simulink model "code_gen"  (Simulink 7.5)
settings: Solver=FixedStepDiscrete  StartTime=0.0  StopTime=10.0  FixedStep=0.001  RelTol=1e-3
InitFcn:
  | boat_constants
values from neighbouring files (symbols this model uses):
  InitialPoint = 0    [boat_constants.m]    (also in l2plus.m)
  IPStar = 0    [boat_constants.m]    (also in l2plus.m)
  ISA_g = 9.815    [boat_constants.m]
  MaxDwnPthStar = 1    [boat_constants.m]    (also in l2plus.m)
  OC2max = 49999    [boat_constants.m]    (also in simulation_constants.m)
  switchDistance = 4    [boat_constants.m]    (also in l2plus.m)
  T_step = 0.01    [boat_constants.m]    (also in common.m)
  tanIntercept = tan( 45*pi/180 )    [boat_constants.m]    (also in l2plus.m)
  TStar = single(4.5)    [boat_constants.m]    (also in l2plus.m = single(2))
  Turn2Track = 0    [boat_constants.m]    (also in l2plus.m)
undefined symbols (not defined in the file or in its folder): buildAndCheckMessage, buildAndCheckSentence, DiscIntNeverNeededParam, ecan1_buffered_transmit_matlab, ecan1_init, getGpsMainData, getSensorData, u1, y1
libraries: simulink x49, dsPICdrivers x22, simulink_need_slupdate x6, microSimulink x4, aerolibconvert2 x3
(part 1 of 3)
settings Model: Creator=bwmairs  LastModifiedBy=bwmairs
settings OptimizationCC: InlineParams=on  InlineInvariantSignals=on  EnhancedBackFolding=on  ZeroExternalMemoryAtStartup=off  ZeroInternalMemoryAtStartup=off  NoFixptDivByZeroProtection=on  EfficientFloat2IntCast=on  OptimizeModelRefInitCode=on
settings DebuggingCC: ReadBeforeWriteMsg=EnableAllAsError  WriteAfterWriteMsg=EnableAllAsError  WriteAfterReadMsg=EnableAllAsError  IntegerOverflowMsg=error  UniqueDataStoreMsg=error
settings HardwareCC: ProdBitPerInt=16  ProdIntDivRoundTo=Zero  ProdEndianess=LittleEndian  ProdWordSize=16  ProdHWDeviceType=16-bit Generic
settings RTWCC: SystemTargetFile=dspic.tlc  TemplateMakefile=dspic_pic30_gcc.tmf  PostCodeGenCommand=dsPIC_Compile()  Description=Embedded Target for Microchip dsPIC (real-time)  ProcessScript=dspic_make_rtw_hook  RTWCompilerOptimization=On
settings RTWCC: CustomSource=|
  | ../../../../ecan/cBuffer.c
  | ../../../../ecan/ecanFunctions.c
  | clib/gps.c
  | clib/sbrk.c
  | clib/commProtocol.c
settings CodeAppCC: IgnoreCustomStorageClasses=off
settings STFCustomTargetCC: IncludeMdlTerminateFcn=off  CombineOutputUpdateFcns=on  SuppressErrorStatus=on  ERTCustomFileBanners=on  SupportNonFinite=off  SupportContinuousTime=off  SupportNonInlinedSFcns=off  SystemTargetFile=dspic.tlc
settings ERTTargetCC: MultiwordLength=2048  ParMdlRefBuildCompliant=off  CompOptLevelCompliant=off  IncludeMdlTerminateFcn=off  SuppressErrorStatus=on  ERTFirstTimeCompliant=off  SupportNonFinite=off  ModelStepFunctionPrototypeControlCompliant=off  CPPClassGenCompliant=off  ExtModeMexFile=noextcomm  InlinedParameterPlacement=NonHierarchical  ERTSrcFileBannerTemplate=dsPIC_code_template.cgt  ERTHdrFileBannerTemplate=dsPIC_code_template.cgt  ERTDataSrcFileTemplate=dsPIC_code_template.cgt  ERTDataHdrFileTemplate=dsPIC_code_template.cgt  ERTCustomFileTemplate=dsPIC_main.tlc
settings CustomProperty: DataType=string  Value=C:\PROGRA~1\MATLAB\R2010a\bin\win32\gmake

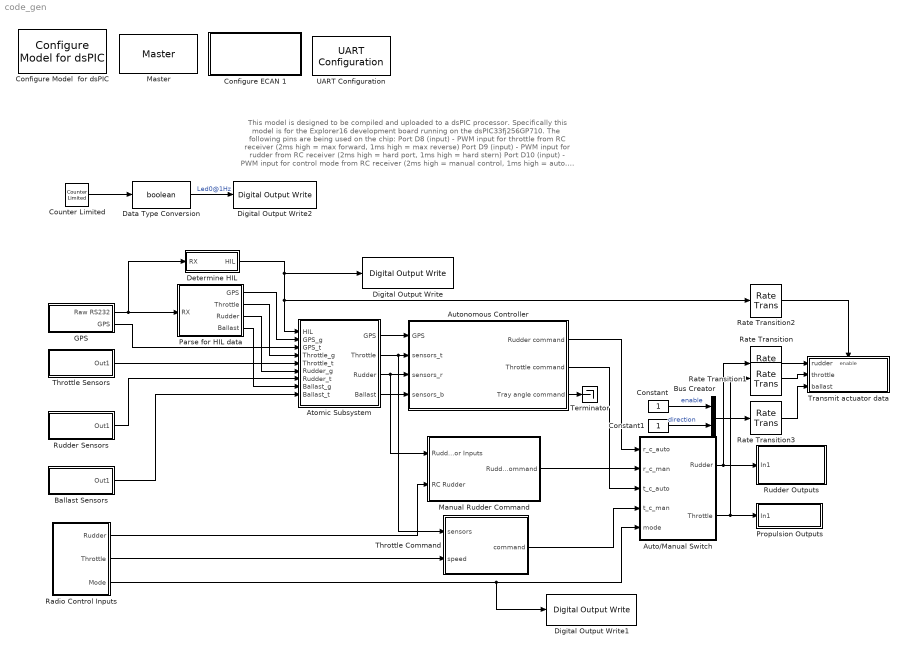
== system code_gen ==
  note: This model is designed to be compiled and uploaded to a dsPIC processor.
      | Specifically this model is for the Explorer16 development board running on
      | the dsPIC33fj256GP710. The following pins are being used on the chip:
      | Port D8 (input) - PWM input for throttle from RC receiver (2ms high = max forward, 1ms high = max reverse)
      | Port D9 (input) - PWM input for rudder from RC receiver (2ms high = hard port, 1ms high = hard stern)
      | Port D10 (input) - PWM input for control mode from RC receiver (2ms high = manual control, 1ms high = auto. control)
      | Port F3 (input) - Port hall effect sensor
      | Port G3 (input) - Starboard hall effect sensor
      | Port B0 (input) - Potentiometer measuring position for the rudder
      | Port OC2/RD1 (output) - Step output for the rudder driver board
      | Port G9 (output) - Enable output for the rudder driver board, wired low
      | Port D5 (output) - Direction output for the rudder driver board (low = rudder turns to port)
      | Ports F0/1 (in/out) - Pins required for the ECAN1 peripheral. This is used for controlling the propeller motor.
      | Ports F4/5 (in/out) - Pins required for the UART2 peripheral. This is used for HIL data or GPS input.
      |
      | A failsafe has been implemented to detect the loss of an RC connection. It reduces propeller speed to zero and
      | disables rudder control.
      |
      | Switching between the autonomous controller and manual control involves using the landing gear channel. When
      | it's enabled, it's under autonomous control. This can only be changed when the RC transmitter is on and connected and
      | is never changed otherwise.
  Atomic Subsystem : Subsystem
  Auto/Manual Switch : Subsystem
  Autonomous Controller : Subsystem
  Ballast Sensors : Subsystem
  Bus Creator : BusCreator  Inputs=2
  Configure ECAN 1 : Subsystem  mask(Initialize ECAN 1){frame_setting=off, mode=Normal, dma_rx_chan=2, dma_tx_chan=0, baud=250000, ps1=8, pd=5, ps2=6, sjw=4, tq=20, triple_sample=on, dma_buf_size=6 buffers, rx_bufs=[], tx_bufs=[0], buf_0_tx_pri=Highest, buf_0_rte=No, buf_1_tx_pri=Highest, buf_1_rte=No, buf_2_tx_pri=Lowest, buf_2_rte=No, buf_3_tx_pri=Lowest, buf_3_rte=No, buf_4_tx_pri=Lowest, buf_4_rte=No, buf_5_tx_pri=Lowest, buf_5_rte=No, buf_6_tx_pri=Lowest, buf_6_rte=No, buf_7_tx_pri=Lowest, buf_7_rte=No, mask_0=0, mask_0_mide=Match std or ext, mask_1=0, mask_1_mide=Match std or ext, mask_2=0, mask_2_mide=Match std or ext, filters=[], filter_0=hex2dec('400'), filter_0_mask=0, filter_0_exide=Match only standard, filter_0_buf=1, filter_1=hex2dec('401'), filter_1_mask=0, filter_1_exide=Match only standard, filter_1_buf=2, filter_2=hex2dec('402'), filter_2_mask=0, filter_2_exide=Match only standard, filter_2_buf=3, filter_3=0, filter_3_mask=0, filter_3_exide=Match only standard, filter_3_buf=0, filter_4=0, filter_4_mask=0, filter_4_exide=Match only standard, filter_4_buf=0, filter_5=0, filter_5_mask=0, filter_5_exide=Match only standard, filter_5_buf=0, filter_6=0, filter_6_mask=0, filter_6_exide=Match only standard, filter_6_buf=0, filter_7=0, filter_7_mask=0, filter_7_exide=Match only standard, filter_7_buf=0, filter_8=0, filter_8_mask=0, filter_8_exide=Match only standard, filter_8_buf=0, filter_9=0, filter_9_mask=<empty>, filter_9_exide=Match only standard, filter_9_buf=0, filter_10=0, filter_10_mask=0, filter_10_exide=Match only standard, filter_10_buf=0, filter_11=0, filter_11_mask=0, filter_11_exide=Match only standard, filter_11_buf=0, filter_12=0, filter_12_mask=0, filter_12_exide=Match only standard, filter_12_buf=0, filter_13=0, filter_13_mask=0, filter_13_exide=Match only standard, filter_13_buf=0, filter_14=0, filter_14_mask=0, filter_14_exide=Match only standard, filter_14_buf=0, filter_15=0, filter_15_mask=0, filter_15_exide=Match only standard, filter_15_buf=0}
      mask prompts: frame_setting "Extended Frames (Standard if unchecked)"; dma_rx_chan "DMA Reception Channel"; dma_tx_chan "DMA Transmission Channel"; baud "Baud Rate (bps)"; ps1 "Phase Segment 1"; pd "Propagation Delay"; ps2 "Phase Segment 2"; sjw "Sync Jump Width"; tq "Time Quanta"; triple_sample "Triple-sample"; dma_buf_size "DMA Buffer Size"; rx_bufs "Reception Buffers"; tx_bufs "Transmission Buffers"; buf_0_tx_pri "Buffer 0 Transmission Priority"; buf_0_rte "Buffer 0 Remote Transmit Enable"; buf_1_tx_pri "Buffer 1 Transmission Priority"; buf_1_rte "Buffer 1 Remote Transmit Enable"; buf_2_tx_pri "Buffer 2 Transmission Priority"; buf_2_rte "Buffer 2 Remote Transmit Enable"; buf_3_tx_pri "Buffer 3 Transmission Priority"; buf_3_rte "Buffer 3 Remote Transmit Enable"; buf_4_tx_pri "Buffer 4 Transmission Priority"; buf_4_rte "Buffer 4 Remote Transmit Enable"; buf_5_tx_pri "Buffer 5 Transmission Priority"; buf_5_rte "Buffer 5 Remote Transmit Enable"; buf_6_tx_pri "Buffer 6 Transmission Priority"; buf_6_rte "Buffer 6 Remote Transmit Enable"; buf_7_tx_pri "Buffer 7 Transmission Priority"; buf_7_rte "Buffer 7 Remote Transmit Enable"; mask_0 "Mask 0"; mask_0_mide "Mask 0 Receive Mode"; mask_1 "Mask 1"; mask_1_mide "Mask 1 Receive Mode"; mask_2 "Mask 2"; mask_2_mide "Mask 2 Receive Mode"; filter_0 "Filter 0"; filter_0_mask "Filter 0 Mask"; filter_0_exide "Filter 0 Mode"; filter_0_buf "Filter 0 Buffer"; filter_1 "Filter 1"; filter_1_mask "Filter 1 Mask"; filter_1_exide "Filter 1 Mode"; filter_1_buf "Filter 1 Buffer"; filter_2 "Filter 2"; filter_2_mask "Filter 2 Mask"; filter_2_exide "Filter 2 Mode"; filter_2_buf "Filter 2 Buffer"; filter_3 "Filter 3"; filter_3_mask "Filter 3 Mask"; filter_3_exide "Filter 3 Mode"; filter_3_buf "Filter 3 Buffer"; filter_4 "Filter 4"; filter_4_mask "Filter 4 Mask"; filter_4_exide "Filter 4 Mode"; filter_4_buf "Filter 4 Buffer"; filter_5 "Filter 5"; filter_5_mask "Filter 5 Mask"; filter_5_exide "Filter 5 Mode"; filter_5_buf "Filter 5 Buffer"; filter_6 "Filter 6"; filter_6_mask "Filter 6 Mask"; filter_6_exide "Filter 6 Mode"; filter_6_buf "Filter 6 Buffer"; filter_7 "Filter 7"; filter_7_mask "Filter 7 Mask"; filter_7_exide "Filter 7 Mode"; filter_7_buf "Filter 7 Buffer"; filter_8 "Filter 8"; filter_8_mask "Filter 8 Mask"; filter_8_exide "Filter 8 Mode"; filter_8_buf "Filter 8 Buffer"; filter_9 "Filter 9"; filter_9_mask "Filter 9 Mask"; filter_9_exide "Filter 9 Mode"; filter_9_buf "Filter 9 Buffer"; filter_10 "Filter 10"; filter_10_mask "Filter 10 Mask"; filter_10_exide "Filter 10 Mode"; filter_10_buf "Filter 10 Buffer"; filter_11 "Filter 11"; filter_11_mask "Filter 11 Mask"; filter_11_exide "Filter 11 Mode"; filter_11_buf "Filter 11 Buffer"; filter_12 "Filter 12"; filter_12_mask "Filter 12 Mask"; filter_12_exide "Filter 12 Mode"; filter_12_buf "Filter 12 Buffer"; filter_13 "Filter 13"; filter_13_mask "Filter 13 Mask"; filter_13_exide "Filter 13 Mode"; filter_13_buf "Filter 13 Buffer"; filter_14 "Filter 14"; filter_14_mask "Filter 14 Mask"; filter_14_exide "Filter 14 Mode"; filter_14_buf "Filter 14 Buffer"; filter_15 "Filter 15"; filter_15_mask "Filter 15 Mask"; filter_15_exide "Filter 15 Mode"; filter_15_buf "Filter 15 Buffer"
      mask help: Initializes the ECAN 1 module on the dsPIC33f. Allows for configuration of almost all ECAN options to produce a usable system.
      mask init:
      | parameters = uint16(zeros(53,1));
      | 
      | %% Generate parameter 1
      | parameters(1) = frame_setting;
      | mode_id = 0;
      | switch mode
      |     case 'Disabled'
      |         mode_id = 1;
      |     case 'Loopback'
      |         mode_id = 2;
      |     case 'Listen only'
      |         mode_id = 3;
      |     case 'Listen all'
      |         mode_id = 7;
      | end
      | parameters(1) = bitor(parameters(1), bitshift(mode_id, 2));
      | parameters(1) = bitor(parameters(1), bitshift(dma_rx_chan, 5));
      | parameters(1) = bitor(parameters(1), bitshift(dma_tx_chan, 8));
      | 
      | %% Generate parameter 2
      | parameters(2) = baud / 100;
      | 
      | %% Generate parameter 3
      | h = find_system(bdroot(gcb),'FollowLinks','on','LookUnderMasks','all','Tag','dsPIC_MASTER');
      | fcy = 0;
      | if ~isempty(h)
      |     %OverrideFcy = strcmp(get_param(h{1},'OverrideFcy'),'on');
      |     %if (OverrideFcy == 1)
      |     %    fcy = str2num(get_param(h{1},'NewFcy'));     %% overridded fcy
      |     %else
      |         fcy = str2num(get_param(h{1},'fcy'));
      |     %end 
      | end
      | parameters(3) = fcy / 1000;
      | 
      | %% Generate parameter 4
      | parameters(4) = ps1 - 1;
      | parameters(4) = bitor(parameters(4), bitshift(pd - 1, 3));
      | parameters(4) = bitor(parameters(4), bitshift(ps2 - 1, 6));
      | parameters(4) = bitor(parameters(4), bitshift(sjw - 1, 9));
      | if triple_sample == 1
      |     parameters(4) = bitset(parameters(4),12);
      | end
      | 
      | %% Generate parameter 5
      | for k = 1:length(filters)
      |     parameters(5) = bitset(parameters(5),filters(k)+1);
      | end;
      | 
      | % Map filter mask values into proper values
      | filter_masks = [filter_0_mask; filter_1_mask; filter_2_mask; filter_3_mask; filter_4_mask; filter_5_mask; filter_6_mask; filter_7_mask; filter_8_mask; filter_9_mask; filter_10_mask; filter_11_mask; filter_12_mask; filter_13_mask; filter_14_mask; filter_15_mask;];
      | filter_masks = filter_masks - 2;
      | filter_masks(filter_masks == -1) = 3;
      | 
      | %% Generate parameters 6 and 7
      | for k = 1:length(filters);
      |     filter = filters(k) + 1;
      |     if filter < 9
      |         parameters(6) = bitor(parameters(6), bitshift(filter_masks(filter),2*(filter-1)));
      |     else
      |         parameters(7) = bitor(parameters(7), bitshift(filter_masks(filter),2*(filter-9)));
      |     end
      | end
      | 
      | % Generate parameters 8 and 9
      | parameters(8) = bitshift(bitand(mask_0,hex2dec('18000000')),-27); % EID17-16
      | parameters(8) = bitor(parameters(8), bitshift(bitand(mask_0,hex2dec('7FF')), 5)); % SID
      | parameters(8) = bitor(parameters(8), bitshift(mask_0_mide - 1, 3)); % MIDE
      | parameters(9) = bitshift(bitand(mask_0,hex2dec('7FFF800')),-11); % EID15-0
      | 
      | %% Generate parameters 10 and 11
      | parameters(10) = bitshift(bitand(mask_1,hex2dec('18000000')),-27); % EID17-16
      | parameters(10) = bitor(parameters(10), bitshift(bitand(mask_1,hex2dec('7FF')), 5)); % SID
      | parameters(10) = bitor(parameters(10), bitshift(mask_1_mide - 1, 3)); % MIDE
      | parameters(11) = bitshift(bitand(mask_1,hex2dec('7FFF800')),-11); % EID15-0
      | 
      | %% Generate parameters 12 and 13
      | parameters(12) = bitshift(bitand(mask_2,hex2dec('18000000')),-27); % EID17-16
      | parameters(12) = bitor(parameters(12), bitshift(bitand(mask_2,hex2dec('7FF')), 5)); % SID
      | parameters(12) = bitor(parameters(12), bitshift(mask_2_mide - 1, 3)); % MIDE
      | parameters(13) = bitshift(bitand(mask_2,hex2dec('7FFF800')),-11); % EID15-0
      | 
      | % Generate parameters 14-17
      | buf_priorities = [buf_0_tx_pri;buf_1_tx_pri;buf_2_tx_pri;buf_3_tx_pri;buf_4_tx_pri;buf_5_tx_pri;buf_6_tx_pri;buf_7_tx_pri] - 1;
      | buf_rtes = [buf_0_rte;buf_1_rte;buf_2_rte;buf_3_rte;buf_4_rte;buf_5_rte;buf_6_rte;buf_7_rte] - 1;
      | 
      | % Create a vector of chars to modify
      | regs = uint16(zeros(8,1));
      | 
      | % Go through all enabled transmission buffers setting appropriate bits
      | for b = 1:size(tx_bufs,1)
      |     
      |     index = tx_bufs(b) + 1;
      |     
      |     % Set transmission bit
      |     regs(index) = bitset(regs(index),8);
      | 
      |     % Set priority bits
      |     regs(index) = bitor(regs(index), buf_priorities(index));
      | 
      |     % Set remote transmit enable bits
      |     if buf_rtes(index) == 1
      |         regs(index) = bitset(regs(index),3);
      |     end
      | end
      | 
      | for b = 1:size(rx_bufs,1)
      |     
      |     index = rx_bufs(b) + 1;
      | 
      |     % Set priority bits
      |     regs(index) = bitor(regs(index), buf_priorities(index));
      | 
      |     % Set remote transmit enable bits
      |     if buf_rtes(index) == 1
      |         regs(index) = bitset(regs(index),3);
      |     end
      | end
      | 
      | % Map our matrix into registers
      | parameters(14) = bitor(bitshift(regs(2),8), regs(1));
      | parameters(15) = bitor(bitshift(regs(4),8), regs(3));
      | parameters(16) = bitor(bitshift(regs(6),8), regs(5));
      | parameters(17) = bitor(bitshift(regs(8),8), regs(7));
      | 
      | % Map the filter buffer values to corresponding bit values
      | filter_buffers = [filter_0_buf; filter_1_buf; filter_2_buf; filter_3_buf; filter_4_buf; filter_5_buf; filter_6_buf; filter_7_buf; filter_8_buf; filter_9_buf; filter_10_buf; filter_11_buf; filter_12_buf; filter_13_buf; filter_14_buf; filter_15_buf;];
      | filter_buffers = filter_buffers - 1;
      | 
      | %% Generate parameter 18
      | if bitget(parameters(5),1) == 1
      |     parameters(18) = filter_buffers(1);
      | end
      | if bitget(parameters(5),2) == 1
      |     parameters(18) = bitor(parameters(18), bitshift(filter_buffers(2), 4));
      | end
      | if bitget(parameters(5),3) == 1
      |     parameters(18) = bitor(parameters(18), bitshift(filter_buffers(3), 8));
      | end
      | if bitget(parameters(5),4) == 1
      |     parameters(18) = bitor(parameters(18), bitshift(filter_buffers(4), 12));
      | end
      | 
      | %% Generate parameter 19
      | if bitget(parameters(5),5) == 1
      |     parameters(19) = filter_buffers(5);
      | end
      | if bitget(parameters(5),6) == 1
      |     parameters(19) = bitor(parameters(19), bitshift(filter_buffers(6), 4));
      | end
      | if bitget(parameters(5),7) == 1
      |     parameters(19) = bitor(parameters(19), bitshift(filter_buffers(7), 8));
      | end
      | if bitget(parameters(5),8) == 1
      |     parameters(19) = bitor(parameters(19), bitshift(filter_buffers(8), 12));
      | end
      | 
      | %% Generate parameter 20
      | if bitget(parameters(5),9) == 1
      |     parameters(20) = filter_buffers(9);
      | end
      | if bitget(parameters(5),10) == 1
      |     parameters(20) = bitor(parameters(20), bitshift(filter_buffers(10), 4));
      | end
      | if bitget(parameters(5),11) == 1
      |     parameters(20) = bitor(parameters(20), bitshift(filter_buffers(11), 8));
      | end
      | if bitget(parameters(5),12) == 1
      |     parameters(20) = bitor(parameters(20), bitshift(filter_buffers(12), 12));
      | end
      | 
      | %% Generate parameter 21
      | if bitget(parameters(5),13) == 1
      |     parameters(21) = filter_buffers(13);
      | end
      | if bitget(parameters(5),14) == 1
      |     parameters(21) = bitor(parameters(21), bitshift(filter_buffers(14), 4));
      | end
      | if bitget(parameters(5),15) == 1
      |     parameters(21) = bitor(parameters(21), bitshift(filter_buffers(15), 8));
      | end
      | if bitget(parameters(5),16) == 1
      |     parameters(21) = bitor(parameters(21), bitshift(filter_buffers(16), 12));
      | end
      | 
      | % Generate parameters 22 and 23
      | parameters(22) = bitshift(bitand(filter_0,hex2dec('18000000')),-27); % EID17-16
      | parameters(22) = bitor(parameters(22), bitshift(bitand(filter_0,hex2dec('7FF')), 5)); % SID
      | parameters(22) = bitor(parameters(22), bitshift(filter_0_exide - 1, 3)); % EXIDE
      | parameters(23) = bitshift(bitand(uint32(filter_0),hex2dec('7FFF800')),-11); % EID15-0
      | 
      | %% Generate parameters 24 and 25
      | parameters(24) = bitshift(bitand(filter_1,hex2dec('18000000')),-27); % EID17-16
      | parameters(24) = bitor(parameters(24), bitshift(bitand(filter_1,hex2dec('7FF')), 5)); % SID
      | parameters(24) = bitor(parameters(24), bitshift(filter_1_exide - 1, 3)); % EXIDE
      | parameters(25) = bitshift(bitand(uint32(filter_1),hex2dec('7FFF800')),-11); % EID15-0
      | 
      | %% Generate parameters 26 and 27
      | parameters(26) = bitshift(bitand(filter_2,hex2dec('18000000')),-27); % EID17-16
      | parameters(26) = bitor(parameters(26), bitshift(bitand(filter_2,hex2dec('7FF')), 5)); % SID
      | parameters(26) = bitor(parameters(26), bitshift(filter_2_exide - 1, 3)); % EXIDE
      | parameters(27) = bitshift(bitand(uint32(filter_2),hex2dec('7FFF800')),-11); % EID15-0
      | 
      | %% Generate parameters 28 and 29
      | parameters(28) = bitshift(bitand(filter_3,hex2dec('18000000')),-27); % EID17-16
      | parameters(28) = bitor(parameters(28), bitshift(bitand(filter_3,hex2dec('7FF')), 5)); % SID
      | parameters(28) = bitor(parameters(28), bitshift(filter_3_exide - 1, 3)); % EXIDE
      | parameters(29) = bitshift(bitand(uint32(filter_3),hex2dec('7FFF800')),-11); % EID15-0
      | 
      | %% Generate parameters 30 and 31
      | parameters(30) = bitshift(bitand(filter_4,hex2dec('18000000')),-27); % EID17-16
      | parameters(30) = bitor(parameters(30), bitshift(bitand(filter_4,hex2dec('7FF')), 5)); % SID
      | parameters(30) = bitor(parameters(30), bitshift(filter_4_exide - 1, 3)); % EXIDE
      | parameters(31) = bitshift(bitand(uint32(filter_4),hex2dec('7FFF800')),-11); % EID15-0
      | 
      | %% Generate parameters 32 and 33
      | parameters(32) = bitshift(bitand(filter_5,hex2dec('18000000')),-27); % EID17-16
      | parameters(32) = bitor(parameters(32), bitshift(bitand(filter_5,hex2dec('7FF')), 5)); % SID
      | parameters(32) = bitor(parameters(32), bitshift(filter_5_exide - 1, 3)); % EXIDE
      | parameters(33) = bitshift(bitand(uint32(filter_5),hex2dec('7FFF800')),-11); % EID15-0
      | 
      | %% Generate parameters 34 and 35
      | parameters(34) = bitshift(bitand(filter_6,hex2dec('18000000')),-27); % EID17-16
      | parameters(34) = bitor(parameters(34), bitshift(bitand(filter_6,hex2dec('7FF')), 5)); % SID
      | parameters(34) = bitor(parameters(34), bitshift(filter_6_exide - 1, 3)); % EXIDE
      | parameters(35) = bitshift(bitand(uint32(filter_6),hex2dec('7FFF800')),-11); % EID15-0
      | 
      | %% Generate parameters 36 and 37
      | parameters(36) = bitshift(bitand(filter_7,hex2dec('18000000')),-27); % EID17-16
      | parameters(36) = bitor(parameters(36), bitshift(bitand(filter_7,hex2dec('7FF')), 5)); % SID
      | parameters(36) = bitor(parameters(36), bitshift(filter_7_exide - 1, 3)); % EXIDE
      | parameters(37) = bitshift(bitand(uint32(filter_7),hex2dec('7FFF800')),-11); % EID15-0
      | 
      | %% Generate parameters 38 and 39
      | parameters(38) = bitshift(bitand(filter_8,hex2dec('18000000')),-27); % EID17-16
      | parameters(38) = bitor(parameters(38), bitshift(bitand(filter_8,hex2dec('7FF')), 5)); % SID
      | parameters(38) = bitor(parameters(38), bitshift(filter_8_exide - 1, 3)); % EXIDE
      | parameters(39) = bitshift(bitand(uint32(filter_8),hex2dec('7FFF800')),-11); % EID15-0
      | 
      | %% Generate parameters 40 and 41
      | parameters(40) = bitshift(bitand(filter_9,hex2dec('18000000')),-27); % EID17-16
      | parameters(40) = bitor(parameters(40), bitshift(bitand(filter_9,hex2dec('7FF')), 5)); % SID
      | parameters(40) = bitor(parameters(40), bitshift(filter_9_exide - 1, 3)); % EXIDE
      | parameters(41) = bitshift(bitand(uint32(filter_9),hex2dec('7FFF800')),-11); % EID15-0
      | 
      | %% Generate parameters 42 and 43
      | parameters(42) = bitshift(bitand(filter_10,hex2dec('18000000')),-27); % EID17-16
      | parameters(42) = bitor(parameters(42), bitshift(bitand(filter_10,hex2dec('7FF')), 5)); % SID
      | parameters(42) = bitor(parameters(42), bitshift(filter_10_exide - 1, 3)); % EXIDE
      | parameters(43) = bitshift(bitand(uint32(filter_10),hex2dec('7FFF800')),-11); % EID15-0
      | 
      | %% Generate parameters 44 and 45
      | parameters(44) = bitshift(bitand(filter_11,hex2dec('18000000')),-27); % EID17-16
      | parameters(44) = bitor(parameters(44), bitshift(bitand(filter_11,hex2dec('7FF')), 5)); % SID
      | parameters(44) = bitor(parameters(44), bitshift(filter_11_exide - 1, 3)); % EXIDE
      | parameters(45) = bitshift(bitand(uint32(filter_11),hex2dec('7FFF800')),-11); % EID15-0
      | 
      | %% Generate parameters 46 and 47
      | parameters(46) = bitshift(bitand(filter_12,hex2dec('18000000')),-27); % EID17-16
      | parameters(46) = bitor(parameters(46), bitshift(bitand(filter_12,hex2dec('7FF')), 5)); % SID
      | parameters(46) = bitor(parameters(46), bitshift(filter_12_exide - 1, 3)); % EXIDE
      | parameters(47) = bitshift(bitand(uint32(filter_12),hex2dec('7FFF800')),-11); % EID15-0
      | 
      | %% Generate parameters 48 and 49
      | parameters(48) = bitshift(bitand(filter_13,hex2dec('18000000')),-27); % EID17-16
      | parameters(48) = bitor(parameters(48), bitshift(bitand(filter_13,hex2dec('7FF')), 5)); % SID
      | parameters(48) = bitor(parameters(48), bitshift(filter_13_exide - 1, 3)); % EXIDE
      | parameters(49) = bitshift(bitand(uint32(filter_13),hex2dec('7FFF800')),-11); % EID15-0
      | 
      | %% Generate parameters 50 and 51
      | parameters(50) = bitshift(bitand(filter_14,hex2dec('18000000')),-27); % EID17-16
      | parameters(50) = bitor(parameters(50), bitshift(bitand(filter_14,hex2dec('7FF')), 5)); % SID
      | parameters(50) = bitor(parameters(50), bitshift(filter_14_exide - 1, 3)); % EXIDE
      | parameters(51) = bitshift(bitand(uint32(filter_14),hex2dec('7FFF800')),-11); % EID15-0
      | 
      | %% Generate parameters 52 and 53
      | parameters(52) = bitshift(bitand(filter_15,hex2dec('18000000')),-27); % EID17-16
      | parameters(52) = bitor(parameters(52), bitshift(bitand(filter_15,hex2dec('7FF')), 5)); % SID
      | parameters(52) = bitor(parameters(52), bitshift(filter_15_exide - 1, 3)); % EXIDE
      | parameters(53) = bitshift(bitand(uint32(filter_15),hex2dec('7FFF800')),-11); % EID15-0
      mask StyleString: checkbox,popup(Disabled|Listen all|Listen only|Loopback|Normal),edit,edit,edit,edit,edit,edit,popup(1|2|3|4),edit,checkbox,popup(4 buffers|6 buffers|8 buffers|12 buffers|16 buffers|24 buffers|32 buffers),edit,edit,popup(Lowest|Low|High|Highest),popup(No|Yes),popup(Lowest|Low|High|Highest),popup(No|Yes),popup(Lowest|Low|High|Highest),popup(No|Yes),popup(Lowest|Low|High|Highest),popup(No|Yes),popup(Lowest|Low|High|Highest),popup(No|Yes),popup(Lowest|Low|High|Highest),popup(No|Yes),popup(Lowest|Low|High|Highest),popup(No|Yes),popup(Lowest|Low|High|Highest),popup(No|Yes),edit,popup(Match std or ext|Obey filter mode),edit,popup(Match std or ext|Obey filter mode),edit,popup(Match std or ext|Obey filter mode),edit,edit,popup(--|0|1|2),popup(Match only standard|Match only extended),popup(0|1|2|3|4|5|6|7|8|9|10|11|12|13|14|FIFO),edit,popup(--|0|1|2),popup(Match only standard|Match only extended),popup(0|1|2|3|4|5|6|7|8|9|10|11|12|13|14|FIFO),edit,popup(--|0|1|2),popup(Match only standard|Match only extended),popup(0|1|2|3|4|5|6|7|8|9|10|11|12|13|14|FIFO),edit,popup(--|0|1|2),popup(Match only standard|Match only extended),popup(0|1|2|3|4|5|6|7|8|9|10|11|12|13|14|FIFO),edit,popup(--|0|1|2),popup(Match only standard|Match only extended),popup(0|1|2|3|4|5|6|7|8|9|10|11|12|13|14|FIFO),edit,popup(--|0|1|2),popup(Match only standard|Match only extended),popup(0|1|2|3|4|5|6|7|8|9|10|11|12|13|14|FIFO),edit,popup(--|0|1|2),popup(Match only standard|Match only extended),popup(0|1|2|3|4|5|6|7|8|9|10|11|12|13|14|FIFO),edit,popup(--|0|1|2),popup(Match only standard|Match only extended),popup(0|1|2|3|4|5|6|7|8|9|10|11|12|13|14|FIFO),edit,popup(--|0|1|2),popup(Match only standard|Match only extended),popup(0|1|2|3|4|5|6|7|8|9|10|11|12|13|14|FIFO),edit,popup(<empty>),popup(Match only standard|Match only extended),popup(0|1|2|3|4|5|6|7|8|9|10|11|12|13|14|FIFO),edit,popup(--|0|1|2),popup(Match only standard|Match only extended),popup(0|1|2|3|4|5|6|7|8|9|10|11|12|13|14|FIFO),edit,popup(--|0|1|2),popup(Match only standard|Match only extended),popup(0|1|2|3|4|5|6|7|8|9|10|11|12|13|14|FIFO),edit,popup(--|0|1|2),popup(Match only standard|Match only extended),popup(0|1|2|3|4|5|6|7|8|9|10|11|12|13|14|FIFO),edit,popup(--|0|1|2),popup(Match only standard|Match only extended),popup(0|1|2|3|4|5|6|7|8|9|10|11|12|13|14|FIFO),edit,popup(--|0|1|2),popup(Match only standard|Match only extended),popup(0|1|2|3|4|5|6|7|8|9|10|11|12|13|14|FIFO),edit,popup(--|0|1|2),popup(Match only standard|Match only extended),popup(0|1|2|3|4|5|6|7|8|9|10|11|12|13|14|FIFO)
      mask CallbackString:
      | |||||tq = 1 + str2num(get_param(gcb, 'ps1')) + str2num(get_param(gcb, 'pd')) + str2num(get_param(gcb, 'ps2'));
      | set_param(gcb, 'tq', int2str(tq));|tq = 1 + str2num(get_param(gcb, 'ps1')) + str2num(get_param(gcb, 'pd')) + str2num(get_param(gcb, 'ps2'));
      | set_param(gcb, 'tq', int2str(tq));|tq = 1 + str2num(get_param(gcb, 'ps1')) + str2num(get_param(gcb, 'pd')) + str2num(get_param(gcb, 'ps2'));
      | set_param(gcb, 'tq', int2str(tq));||||||filters = eval(get_param(gcb,'tx_bufs'));
      | mVisibilities = get_param(gcb,'MaskVisibilities');
      | mNames = get_param(gcb,'MaskNames');
      | for i = 1:size(mNames);
      | 	n = mNames{i};
      |     if size(n,2) > 4 && strcmp(n(1:4), 'buf_') == 1
      |         filterNumber = sscanf(n, 'buf_%d');
      |         if isempty(find(filters == filterNumber, 1)) == 0
      |              mVisibilities{i} = 'on';
      |         else
      |              mVisibilities{i} = 'off';
      |         end
      |     end
      | end
      | set_param(gcb, 'MaskVisibilities', mVisibilities);|||||||||||||||||||||||filters = eval(get_param(gcb,'filters'));
      | mVisibilities = get_param(gcb,'MaskVisibilities');
      | mNames = get_param(gcb,'MaskNames');
      | for i = 1:size(mNames);
      | 	n = mNames{i};
      |     if size(n,2) > 7 && strcmp(n(1:7), 'filter_') == 1
      |         filterNumber = sscanf(n, 'filter_%d');
      |         if isempty(find(filters == filterNumber, 1)) == 0
      |              mVisibilities{i} = 'on';
      |         else
      |              mVisibilities{i} = 'off';
      |         end
      |     end
      | end
      | set_param(gcb, 'MaskVisibilities', mVisibilities);||||||||||||||||||||||||||||||||||||||||||||||||||||||||||||||||
      mask Display: text(0.5,0.5,'Configure ECAN1','horizontalAlignment','center','verticalAlignment','middle');
  Configure Model  for dsPIC : dsPICdrivers/Simulink Configuration/Configure Model  for dsPIC
  Constant : Constant  OutDataTypeMode=boolean  OutDataType=fixdt(1, 16)  OutScaling=2^0  OutDataTypeStr=boolean
  Constant1 : Constant  OutDataTypeMode=boolean  OutDataType=fixdt(1, 16)  OutScaling=2^0  OutDataTypeStr=boolean
  Counter Limited : simulink/Sources/Counter Limited  SystemSampleTime=-1  uplimit=1  tsamp=1
  Data Type Conversion : DataTypeConversion  OutDataTypeMode=boolean  OutDataType=sfix(16)  OutScaling=2^0  OutDataTypeStr=boolean
  Determine HIL : Subsystem
  Digital Output Write : dsPICdrivers/Digital I//O/Digital Output Write  Tag=dsPIC_Digital_Output  Priority=5  PORT=A  Pin=[1]  Simultaneous=off  OrderingInOutPopup=None
  Digital Output Write1 : dsPICdrivers/Digital I//O/Digital Output Write  Tag=dsPIC_Digital_Output  Priority=5  PORT=A  Pin=[2]  Simultaneous=off  OrderingInOutPopup=None
  Digital Output Write2 : dsPICdrivers/Digital I//O/Digital Output Write  Tag=dsPIC_Digital_Output  Priority=5  PORT=A  Pin=[7]  Simultaneous=off  OrderingInOutPopup=None
  GPS : Subsystem
  Manual Rudder Command : Subsystem
  Master : dsPICdrivers/Master  Tag=dsPIC_MASTER  Priority=1  TimeStepType=Timer1  picType=33fJ256GP710  fcy=40000000  Quartz_33f=8e6  PLLActive_33f=on  fcyDesired_33f=40000000  tmr1="[1  39999  0]"  tmr1Info="Time Step : 0.001  ;   Error : 0%  PR1=39999"  tmr2345="[8  0  0  0  0  0  0  0]"  tmr2345cfg=[-1 -1 -1 -1 -1 -1 -1 -1]  IOautoConf=on  typePort="[ 10  10  10   0   0   0   0  10   0   0   0   0   0   0   0   0   8   0   0   0   0   0   0   0   0   0   0   0   0   0   0   0   0   0   0   0   0   0   0   0   0   0   0   0   0   0   0   0   0   7   0   0   0  10   0   0   0   6   6   6   0   0   0   0   0   0   0   0   0   0   0   0   0   0   0   0   0   0   0   0   0   0   0   9   4   5   0   0   0   0   0   0   0   0   0   0   0   0   0   9   0   0   0   0   0  10   0   0   0   0   0   0 ]"  TRIS="[ 65400  65535  65535  65501  65535  65535  65023 ]"  ADPCFG=8388608  MasterBusyPort=None  MasterOverloadPort=None  FOSC=Quartz (XT - HS)  ClockSwitchMonitor=Both disabled  TempProtection_33f=TEMP_ON  FPBOR=<empty>  PWRT=disable  MCLR=<empty>  ICD=ICS_NONE  JTAGEN=JTAGEN_OFF  PowerSave=off  OverrideFcy=off  NewFcy=1e6  PR2345="[65535  65535  65535  65535  65535  65535  65535  65535]"
  Parse for HIL data : Subsystem
  Propulsion Outputs : Subsystem
  Radio Control Inputs : Subsystem
  Rate Transition{,1..3} (4 alike) : RateTransition  OutPortSampleTime=1
  Rudder Outputs : Subsystem
  Rudder Sensors : Subsystem
  Terminator : Terminator
  Throttle Command : Subsystem
  Throttle Sensors : Subsystem
  Transmit actuator data : Subsystem  TreatAsAtomicUnit=on
  UART Configuration : dsPICdrivers/Serial PORT/UART Configuration  Tag=dsPIC_config_UART  Priority=2  UART=2  proposed_BAUD=1200  ALT_TX_RX=on  InterruptTxWhen=Do not use interrupt  TXInterruptPri=2  TxBufferSize=128  TXEN=on  InterruptRxWhen=When a character is received  RXInterruptPri=1  RxBufferSize=128  BAUD=1200  UxBRG=2082  Info="UxBRG = 2082   ||  Real Baud : 1200   ||  % error : 0.016003  ||  max 0.12002 Bytes / Step"  RealBaud=0
  wires:
  Rudder Sensors/1(Out1) -> Atomic Subsystem/7(Rudder_t)
  Radio Control Inputs/1(Rudder) -> Manual Rudder Command/2(RC Rudder)
  Autonomous Controller/1(Rudder command) -> Auto/Manual Switch/1(r_c_auto)
  Manual Rudder Command/1(Rudder Command) -> Auto/Manual Switch/2(r_c_man)
  Autonomous Controller/2(Throttle command) -> Auto/Manual Switch/3(t_c_auto)
  Auto/Manual Switch/2(Throttle) -> Propulsion Outputs/1(In1), Rate Transition1/1
  Radio Control Inputs/3(Mode) -> Auto/Manual Switch/5(mode), Digital Output Write1/1
  Auto/Manual Switch/1(Rudder) -> Rudder Outputs/1(In1), Rate Transition/1
  GPS/1(Raw RS232) -> Determine HIL/1(RX), Parse for HIL data/1(RX)
  Atomic Subsystem/1(GPS) -> Autonomous Controller/1(GPS)
  Atomic Subsystem/2(Throttle) -> Autonomous Controller/2(sensors_t), Throttle Command/1(sensors)
  Atomic Subsystem/3(Rudder) -> Autonomous Controller/3(sensors_r), Manual Rudder Command/1(Rudder Sensor Inputs)
  Atomic Subsystem/4(Ballast) -> Autonomous Controller/4(sensors_b)
  Determine HIL/1(HIL) -> Digital Output Write/1, Atomic Subsystem/1(HIL), Rate Transition2/1
  GPS/2(GPS) -> Atomic Subsystem/3(GPS_t)
  Throttle Sensors/1(Out1) -> Atomic Subsystem/5(Throttle_t)
  Ballast Sensors/1(Out1) -> Atomic Subsystem/9(Ballast_t)
  Parse for HIL data/1(GPS) -> Atomic Subsystem/2(GPS_g)
  Parse for HIL data/2(Throttle) -> Atomic Subsystem/4(Throttle_g)
  Parse for HIL data/3(Rudder) -> Atomic Subsystem/6(Rudder_g)
  Parse for HIL data/4(Ballast) -> Atomic Subsystem/8(Ballast_g)
  Radio Control Inputs/2(Throttle) -> Throttle Command/2(speed)
  Throttle Command/1(command) -> Auto/Manual Switch/4(t_c_man)
  Counter Limited/1 -> Data Type Conversion/1
  Data Type Conversion/1 -> Digital Output Write2/1  "Led0@1Hz"
  Rate Transition/1 -> Transmit actuator data/1(rudder)
  Rate Transition1/1 -> Transmit actuator data/2(throttle)
  Rate Transition2/1 -> Transmit actuator data/Enable
  Autonomous Controller/3(Tray angle command) -> Terminator/1
  Rate Transition3/1 -> Transmit actuator data/3(ballast)
  Constant/1 -> Bus Creator/1  "enable"
  Bus Creator/1 -> Rate Transition3/1
  Constant1/1 -> Bus Creator/2  "direction"

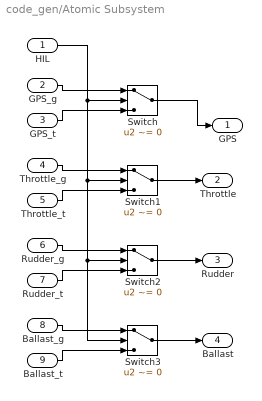
== system code_gen/Atomic Subsystem ==
  HIL : Inport  OutDataType=fixdt(1, 16)  OutScaling=2^0
  GPS_g : Inport  Port=2  OutDataType=fixdt(1, 16)  OutScaling=2^0
  GPS_t : Inport  Port=3  OutDataType=fixdt(1, 16)  OutScaling=2^0
  Throttle_g : Inport  Port=4  OutDataType=fixdt(1, 16)  OutScaling=2^0
  Throttle_t : Inport  Port=5  OutDataType=fixdt(1, 16)  OutScaling=2^0
  Rudder_g : Inport  Port=6  OutDataType=fixdt(1, 16)  OutScaling=2^0
  Rudder_t : Inport  Port=7  OutDataType=fixdt(1, 16)  OutScaling=2^0
  Ballast_g : Inport  Port=8  OutDataType=fixdt(1, 16)  OutScaling=2^0
  Ballast_t : Inport  Port=9  OutDataType=fixdt(1, 16)  OutScaling=2^0
  Switch{,1..3} (4 alike) : Switch  Criteria=u2 ~= 0  OutDataType=fixdt(1, 16)  OutScaling=2^0
  GPS : Outport  OutDataType=fixdt(1, 16)  OutScaling=2^0
  Throttle : Outport  Port=2  OutDataType=fixdt(1, 16)  OutScaling=2^0
  Rudder : Outport  Port=3  OutDataType=fixdt(1, 16)  OutScaling=2^0
  Ballast : Outport  Port=4  OutDataType=fixdt(1, 16)  OutScaling=2^0
  wires:
  HIL/1 -> Switch/2, Switch1/2, Switch2/2, Switch3/2
  GPS_g/1 -> Switch/1
  GPS_t/1 -> Switch/3
  Switch/1 -> GPS/1
  Throttle_g/1 -> Switch1/1
  Throttle_t/1 -> Switch1/3
  Switch1/1 -> Throttle/1
  Rudder_g/1 -> Switch2/1
  Rudder_t/1 -> Switch2/3
  Switch2/1 -> Rudder/1
  Ballast_g/1 -> Switch3/1
  Ballast_t/1 -> Switch3/3
  Switch3/1 -> Ballast/1

== system code_gen/Auto/Manual Switch ==
  r_c_auto : Inport
  r_c_man : Inport  Port=2
  t_c_auto : Inport  Port=3
  t_c_man : Inport  Port=4
  mode : Inport  Port=5
  Switch1 : Switch  Criteria=u2 ~= 0  Threshold=1  OutDataType=fixdt(1, 16)  OutScaling=2^0
  Switch5 : Switch  Threshold=1  OutDataType=fixdt(1, 16)  OutScaling=2^0
  Rudder : Outport
  Throttle : Outport  Port=2
  wires:
  t_c_auto/1 -> Switch1/1
  Switch1/1 -> Throttle/1
  t_c_man/1 -> Switch1/3
  r_c_man/1 -> Switch5/3
  Switch5/1 -> Rudder/1  "enable"
  mode/1 -> Switch1/2, Switch5/2
  r_c_auto/1 -> Switch5/1

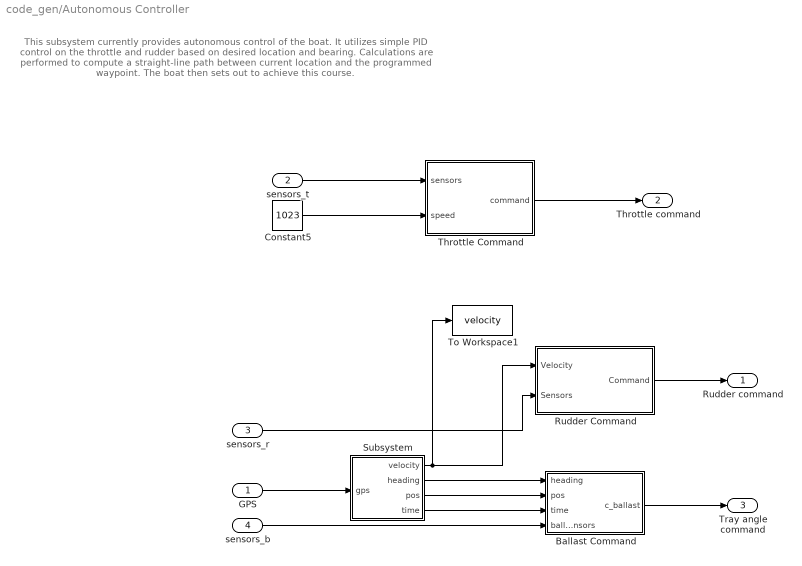
== system code_gen/Autonomous Controller ==
  note: This subsystem currently provides autonomous control of the boat. It utilizes simple PID control
      | on the throttle and rudder based on desired location and bearing. Calculations are performed
      | to compute a straight-line path between current location and the programmed waypoint. The
      | boat then sets out to achieve this course.
  GPS : Inport  OutDataType=sfix(16)  OutScaling=2^0
  sensors_t : Inport  Port=2  OutDataType=sfix(16)  OutScaling=2^0
  sensors_r : Inport  Port=3  OutDataType=sfix(16)  OutScaling=2^0
  sensors_b : Inport  Port=4  OutDataType=sfix(16)  OutScaling=2^0
  Ballast Command : Subsystem
  Constant5 : Constant  Value=1023  OutDataTypeMode=int16  OutDataType=sfix(16)  OutScaling=2^0  OutDataTypeStr=int16
  Rudder Command : Subsystem
  Subsystem : Subsystem
  Throttle Command : Subsystem
  To Workspace1 : ToWorkspace  VariableName=velocity  SampleTime=-1  SaveFormat=Array
  Rudder command : Outport  OutDataType=sfix(16)  OutScaling=2^0
  Throttle command : Outport  Port=2  OutDataType=sfix(16)  OutScaling=2^0
  Tray angle command : Outport  Port=3  OutDataType=sfix(16)  OutScaling=2^0
  wires:
  Throttle Command/1(command) -> Throttle command/1
  Constant5/1 -> Throttle Command/2(speed)
  Rudder Command/1(Command) -> Rudder command/1
  GPS/1 -> Subsystem/1(gps)
  Ballast Command/1(c_ballast) -> Tray angle command/1
  sensors_b/1 -> Ballast Command/4(ballast sensors)
  sensors_r/1 -> Rudder Command/2(Sensors)
  sensors_t/1 -> Throttle Command/1(sensors)
  Subsystem/2(heading) -> Ballast Command/1(heading)
  Subsystem/3(pos) -> Ballast Command/2(pos)
  Subsystem/4(time) -> Ballast Command/3(time)
  Subsystem/1(velocity) -> Rudder Command/1(Velocity), To Workspace1/1

== system code_gen/Ballast Sensors ==
  Bus Creator : BusCreator  Inputs=3
  Constant : Constant  Value=0  OutDataTypeMode=uint16  OutDataType=fixdt(1, 16)  OutScaling=2^0  OutDataTypeStr=uint16  SampleTime=T_step
  Constant1 : Constant  Value=0  OutDataTypeMode=boolean  OutDataType=fixdt(1, 16)  OutScaling=2^0  OutDataTypeStr=boolean  SampleTime=T_step
  Constant2 : Constant  Value=0  OutDataTypeMode=boolean  OutDataType=fixdt(1, 16)  OutScaling=2^0  OutDataTypeStr=boolean  SampleTime=T_step
  Out1 : Outport
  wires:
  Bus Creator/1 -> Out1/1
  Constant2/1 -> Bus Creator/3  "limit port"
  Constant1/1 -> Bus Creator/2  "limit starboard"
  Constant/1 -> Bus Creator/1  "position"

== system code_gen/Configure ECAN 1 ==
  C Function Call [ecanFunctions.c] : dsPICdrivers/OTHERS/C Function Call  Tag=dsPIC_dsPIC_CFunctionCall  fctName='ecan1_init'  INPUT_SIZE=53  INPUT1=uint16  INPUT2=--  INPUT3=--  OUTPUT_SIZE=1  OUTPUT1=--  SampleTime=Inf  InputType=[ 4 ]  OutputType=[ ]  FctDeclaration=extern void ecan1_init(uint16_T* u1);  FctCall=ecan1_init(*%u1);  OrderingInOutPopup=None
  Constant : Constant  Value=parameters  OutDataTypeMode=uint16  OutDataType=sfix(16)  OutScaling=2^0  OutDataTypeStr=uint16
  wires:
  Constant/1 -> C Function Call [ecanFunctions.c]/1

== system code_gen/Determine HIL ==
  RX : Inport
  Compare To Constant : simulink/Logic and Bit Operations/Compare To Constant  SystemSampleTime=-1  relop===  const=5  LogicOutDataTypeMode=uint8
  Compare To Constant1 : simulink/Logic and Bit Operations/Compare To Constant  SystemSampleTime=-1  relop=>=  const=.05  LogicOutDataTypeMode=boolean
  Discrete-Time Integrator : DiscreteIntegrator  InitialConditionMode=State only (most efficient)  SampleTime=-1  OutDataType=fixdt(1, 16)  OutScaling=2^0  OutDataTypeStr=Inherit: Inherit via back propagation  LimitOutput=on  UpperSaturationLimit=5  LowerSaturationLimit=0  ICPrevOutput=DiscIntNeverNeededParam  ICPrevScaledInput=DiscIntNeverNeededParam
  HIL : Outport
  wires:
  Compare To Constant/1 -> Discrete-Time Integrator/1
  Discrete-Time Integrator/1 -> Compare To Constant1/1
  RX/1 -> Compare To Constant/1
  Compare To Constant1/1 -> HIL/1

== system code_gen/GPS ==
  Bus Creator : BusCreator  Inputs=11
  C Function Call : dsPICdrivers/OTHERS/C Function Call  Tag=dsPIC_dsPIC_CFunctionCall  fctName='buildAndCheckSentence'  INPUT_SIZE=1  INPUT1=uint8  INPUT2=--  INPUT3=--  OUTPUT_SIZE=1  OUTPUT1=--  SampleTime=-1  InputType=[ 2 ]  OutputType=[ ]  FctDeclaration=extern void buildAndCheckSentence(uint8_T u1);  FctCall=buildAndCheckSentence(%u1);  OrderingInOutPopup=None
  Demux : Demux  Outputs=7
  Digital Output Write : dsPICdrivers/Digital I//O/Digital Output Write  Tag=dsPIC_Digital_Output  Priority=5  PORT=A  Pin=[0]  Simultaneous=off  OrderingInOutPopup=None
  Embedded MATLAB Function : Stateflow chart  TreatAsAtomicUnit=on
  Embedded MATLAB Function1 : Stateflow chart  TreatAsAtomicUnit=on
  Produce the GPS Main Data and update the AP State (lat lon hei cog sog ddmmyy hhmmss) [gps.c] : dsPICdrivers/OTHERS/C Function Call  Tag=dsPIC_dsPIC_CFunctionCall  fctName='getGpsMainData'  INPUT_SIZE=1  INPUT1=--  INPUT2=--  INPUT3=--  OUTPUT_SIZE=7  OUTPUT1=real32  SampleTime=.01  InputType=[ ]  OutputType=[ 7 ]  FctDeclaration=extern void getGpsMainData(real32_T* y1);  FctCall=getGpsMainData(*%y1);  OrderingInOutPopup=None
  Rx Input : dsPICdrivers/Serial PORT/Rx Input  Tag=dsPIC_RX  Priority=5  UART=2  SampleTime=.01  BlockingFctChk=off  OutputDefault=0  IsPresentFlagChk=on
  Raw RS232 : Outport
  GPS : Outport  Port=2
  wires:
  Produce the GPS Main Data and update the AP State (lat lon hei cog sog ddmmyy hhmmss) [gps.c]/1 -> Demux/1
  Bus Creator/1 -> GPS/1
  Demux/3 -> Bus Creator/3  "altitude"
  Demux/2 -> Bus Creator/2  "longitude"
  Demux/1 -> Bus Creator/1  "latitude"
  Rx Input/2 -> Digital Output Write/1
  Rx Input/1 -> C Function Call/1, Raw RS232/1
  Demux/5 -> Embedded MATLAB Function1/1(u)
  Demux/4 -> Embedded MATLAB Function/1(u)
  Embedded MATLAB Function1/3(c) -> Bus Creator/9  "second"
  Embedded MATLAB Function1/2(b) -> Bus Creator/8  "minute"
  Embedded MATLAB Function1/1(a) -> Bus Creator/7  "hour"
  Embedded MATLAB Function/3(c) -> Bus Creator/6  "day"
  Embedded MATLAB Function/2(b) -> Bus Creator/5  "month"
  Embedded MATLAB Function/1(a) -> Bus Creator/4  "year"
  Demux/6 -> Bus Creator/10  "cog"
  Demux/7 -> Bus Creator/11  "sog"

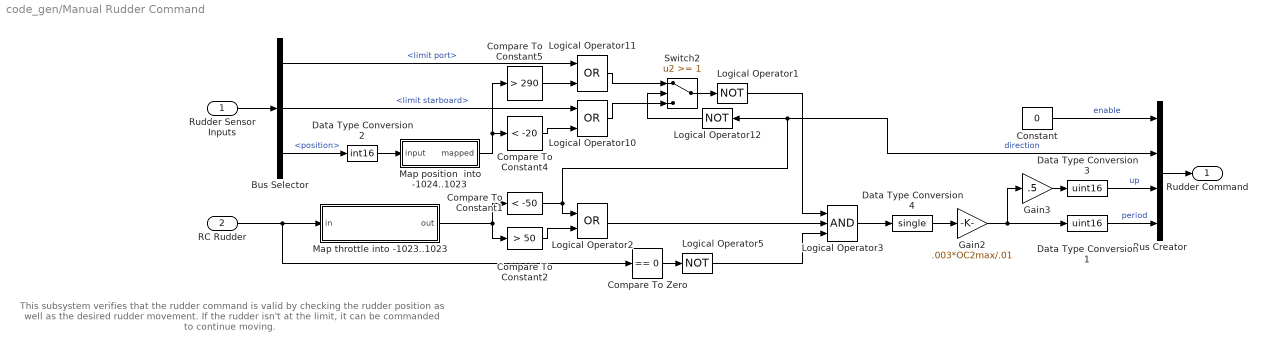
== system code_gen/Manual Rudder Command ==
  note: This subsystem verifies that the rudder command is valid by checking the
      | rudder position as well as the desired rudder movement. If the rudder isn't
      | at the limit, it can be commanded to continue moving.
  Rudder Sensor Inputs : Inport  OutDataType=sfix(16)  OutScaling=2^0
  RC Rudder : Inport  Port=2  OutDataType=sfix(16)  OutScaling=2^0
  Bus Creator : BusCreator
  Bus Selector : BusSelector  OutputSignals=limit port,limit starboard,position
  Compare To Constant1 : simulink/Logic and Bit Operations/Compare To Constant  SystemSampleTime=-1  relop=<  const=-50  LogicOutDataTypeMode=boolean  ZeroCross=off
  Compare To Constant2 : simulink/Logic and Bit Operations/Compare To Constant  SystemSampleTime=-1  relop=>  const=50  LogicOutDataTypeMode=boolean  ZeroCross=off
  Compare To Constant4 : simulink/Logic and Bit Operations/Compare To Constant  SystemSampleTime=-1  relop=<  const=-20  LogicOutDataTypeMode=boolean  ZeroCross=off
  Compare To Constant5 : simulink/Logic and Bit Operations/Compare To Constant  SystemSampleTime=-1  relop=>  const=290  LogicOutDataTypeMode=boolean  ZeroCross=off
  Compare To Zero : simulink/Logic and Bit Operations/Compare To Zero  SystemSampleTime=-1  relop===  LogicOutDataTypeMode=boolean  ZeroCross=off
  Constant : Constant  Value=0  OutDataTypeMode=boolean  OutDataType=sfix(16)  OutScaling=2^0  OutDataTypeStr=boolean
  Data Type Conversion1 : DataTypeConversion  OutDataTypeMode=uint16  OutDataType=sfix(16)  OutScaling=2^0  OutDataTypeStr=uint16  RndMeth=Simplest
  Data Type Conversion2 : DataTypeConversion  OutDataTypeMode=int16  OutDataType=sfix(16)  OutScaling=2^0  OutDataTypeStr=int16
  Data Type Conversion3 : DataTypeConversion  OutDataTypeMode=uint16  OutDataType=sfix(16)  OutScaling=2^0  OutDataTypeStr=uint16  RndMeth=Simplest
  Data Type Conversion4 : DataTypeConversion  OutDataTypeMode=single  OutDataType=sfix(16)  OutScaling=2^0  OutDataTypeStr=single
  Gain2 : Gain  Gain=.003*OC2max/.01  ParameterDataType=sfix(16)  ParameterScaling=2^0  OutDataType=sfix(16)  OutScaling=2^0  OutDataTypeStr=Inherit: Same as input
  Gain3 : Gain  Gain=.5  ParameterDataType=sfix(16)  ParameterScaling=2^0  OutDataType=sfix(16)  OutScaling=2^0  OutDataTypeStr=Inherit: Same as input
  Logical Operator1 : Logic  Operator=NOT  AllPortsSameDT=off  OutDataTypeMode=boolean  OutDataTypeStr=boolean
  Logical Operator10 : Logic  Operator=OR  AllPortsSameDT=off  OutDataTypeMode=boolean  OutDataTypeStr=boolean
  Logical Operator11 : Logic  Operator=OR  AllPortsSameDT=off  OutDataTypeMode=boolean  OutDataTypeStr=boolean
  Logical Operator12 : Logic  Operator=NOT  AllPortsSameDT=off  OutDataTypeMode=boolean  OutDataTypeStr=boolean
  Logical Operator2 : Logic  Operator=OR  AllPortsSameDT=off  OutDataTypeMode=boolean  OutDataTypeStr=boolean
  Logical Operator3 : Logic  Inputs=3  AllPortsSameDT=off  OutDataTypeMode=Specify via dialog  OutDataTypeStr=uint(8)
  Logical Operator5 : Logic  Operator=NOT  AllPortsSameDT=off  OutDataTypeMode=boolean  OutDataTypeStr=boolean
  Map position  into -1024..1023 : Subsystem
  Map throttle into -1023..1023 : Subsystem
  Switch2 : Switch  Threshold=1  OutDataTypeStr=Inherit: Inherit via back propagation
  Rudder Command : Outport
  wires:
  Compare To Constant2/1 -> Logical Operator2/2
  Logical Operator2/1 -> Logical Operator3/2
  Logical Operator12/1 -> Switch2/2
  Switch2/1 -> Logical Operator1/1
  Logical Operator10/1 -> Switch2/3
  Logical Operator11/1 -> Switch2/1
  Logical Operator3/1 -> Data Type Conversion4/1
  Logical Operator1/1 -> Logical Operator3/1
  Data Type Conversion2/1 -> Map position  into -1024..1023/1(input)
  Map position  into -1024..1023/1(mapped) -> Compare To Constant5/1, Compare To Constant4/1
  Map throttle into -1023..1023/1(out) -> Compare To Constant1/1, Compare To Constant2/1
  Compare To Constant5/1 -> Logical Operator11/2
  Compare To Constant4/1 -> Logical Operator10/2
  Logical Operator5/1 -> Logical Operator3/3
  Compare To Zero/1 -> Logical Operator5/1
  Data Type Conversion4/1 -> Gain2/1
  Compare To Constant1/1 -> Logical Operator12/1, Bus Creator/2, Logical Operator2/1  "direction"
  Gain2/1 -> Gain3/1, Data Type Conversion1/1
  RC Rudder/1 -> Compare To Zero/1, Map throttle into -1023..1023/1(in)
  Rudder Sensor Inputs/1 -> Bus Selector/1
  Gain3/1 -> Data Type Conversion3/1
  Bus Creator/1 -> Rudder Command/1
  Bus Selector/2 -> Logical Operator10/1  "<limit starboard>"
  Bus Selector/1 -> Logical Operator11/1  "<limit port>"
  Bus Selector/3 -> Data Type Conversion2/1  "<position>"
  Data Type Conversion1/1 -> Bus Creator/4  "period"
  Data Type Conversion3/1 -> Bus Creator/3  "up"
  Constant/1 -> Bus Creator/1  "enable"
